simulink model "ADRC_IM"  (R2023b)
settings: Solver=FixedStepAuto  StartTime=0  StopTime=5  FixedStep=Ts  RelTol=1e-3
InitFcn:
  | Parameters_v7_1;
  | Parameters;
  | Sim;
StartFcn:
  | Parameters_v7_1;
  | Parameters;
  | Sim;
values from neighbouring files (symbols this model uses):
  F = 0.01    [Parameters_v7_2.m]
  J = 1.662    [Parameters_v7_2.m]
  ki_m = ((wc_m^2)*J)/(Kt)    [Parameters.m]
  kp_m = (2*damp*wc_m*J-F)/Kt    [Parameters.m]
  kr = Lm/Lr    (= 0.977464788732)    [Parameters_v7_2.m]
  Lm = 34.7e-3    (= 0.0347)    [Parameters_v7_2.m]
  p = 2    [Parameters_v7_2.m]
  r_sigma = Rs+kr^2*Rr    (= 0.304839730212)    [Parameters_v7_2.m]
  Rs = 0.087    [Parameters_v7_2.m]
  sf_nom = 0.973    [Parameters.m]    (also in Parameters_v7_2.m = 0.9)
  T_nom = 229    [Parameters_v7_2.m]
  t_sigma = sigma*Ls/r_sigma    (= 0.00518951984994)    [Parameters_v7_2.m]
  tr = Lr/Rr    (= 0.155701754386)    [Parameters_v7_2.m]
  Ts = 1e-6    (= 1e-06)    [Parameters.m]    (also in Parameters_v7_2.m = 5e-05)
  Tss = 1/fr    (= 2.5e-05)    [Parameters.m]
  Vdc = 780    [Parameters_v7_2.m]
undefined symbols (not defined in the file or in its folder): DiscIntNeverNeededParam, sigbuilder_block
libraries: spsAlphaBetaZerotoabcLib x2, slctrl_adaptive x1, slpidlib x1, spspowerguiLib x1
settings Model: Creator=Alvaro  LastModifiedBy=Selim
settings DebuggingCC: UnconnectedInputMsg=warning  UnconnectedOutputMsg=warning  UnconnectedLineMsg=warning
settings ModelReferenceCC: EnableRefExpFcnMdlSchedulingChecks=on
settings RTWCC: DLArmComputeVersion=19.05

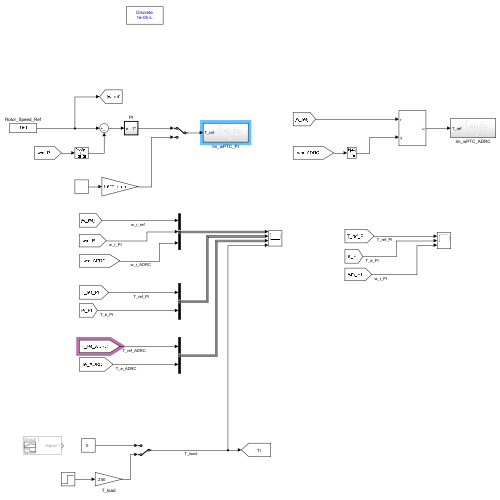
[thumbnail: Simulink's stored preview of the top-level diagram]
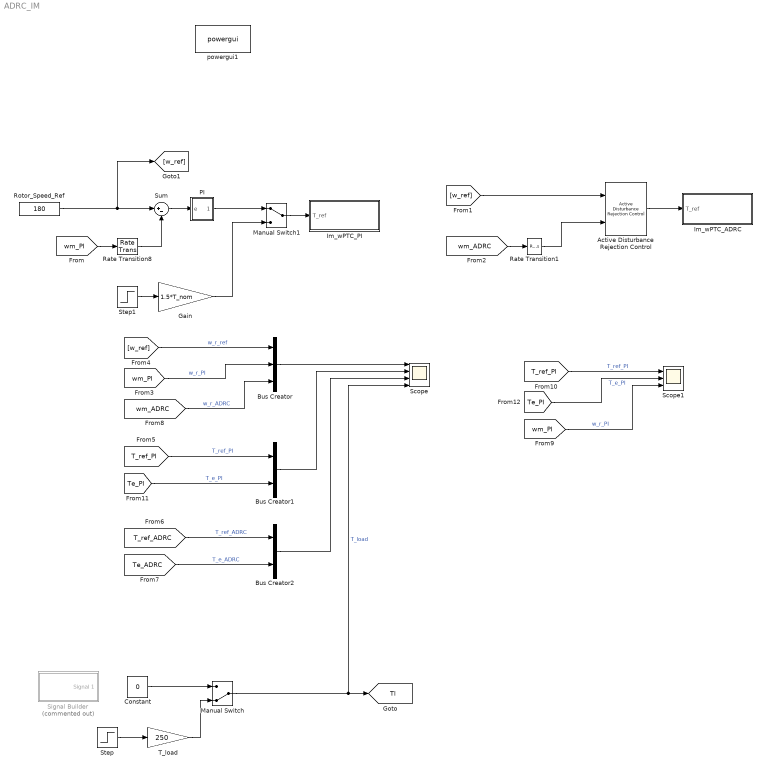
== system ADRC_IM ==
  Active Disturbance Rejection Control : slctrl_adaptive/Active Disturbance Rejection Control  time_domain=discrete-time  Ts=Ts  model_type=second-order  b0=b  wc=omega_C  wo=omega_O  x0=0  ulim_checkbox=on  umax=T_nom*1.5  umin=-T_nom*1.5  xhat_checkbox=off
      settings: LibrarySourceBlock=slctrlblks/Adaptive Control/Active Disturbance Rejection Control
  Bus Creator : BusCreator  Inputs=3
  Bus Creator1 : BusCreator  Inputs=2
  Bus Creator2 : BusCreator  Inputs=2
  Constant : Constant  Value=0
  Gain : Gain  Gain=1.5*T_nom
  Im_wPTC_ADRC : Subsystem
  Im_wPTC_PI : Subsystem
  Manual Switch : ManualSwitch  CurrentSetting=0
  Manual Switch1 : ManualSwitch
  PI : Subsystem  TreatAsAtomicUnit=on  SystemSampleTime=Tss
  Rate Transition1 : RateTransition  Integrity=off  Deterministic=off  InitialCondition=120  OutPortSampleTime=Ts
  Rate Transition8 : RateTransition  Integrity=off  Deterministic=off  InitialCondition=120  OutPortSampleTime=Ts
  Rotor_Speed_Ref : Constant  Value=180
  Scope : Scope  NumInputPorts=4
  Scope1 : Scope  NumInputPorts=3
  Signal Builder : Subsystem  Tag=STV Subsys  Commented=on  LoadFcn=sigbuilder_block('load');  StartFcn=sigbuilder_block('start');  StopFcn=sigbuilder_block('stop');  ClipboardFcn=sigbuilder_block('clipboard');  mask(Sigbuilder block){tuvar=[0:10]}
      mask help: Simulink:masks:SigbuilderBlock_MD
      mask init:
      | if ~strcmp(get_param(bdroot(gcbh),'SimulationStatus'),'stopped') tuvar = sigbuilder_block('maskInit'); end
      settings: CopyFcn=sigbuilder_block('copy');  DeleteFcn=sigbuilder_block('delete');  ModelCloseFcn=sigbuilder_block('modelClose');  PreSaveFcn=sigbuilder_block('preSave');  PauseFcn=sigbuilder_block('pause');  ContinueFcn=sigbuilder_block('continue');  NameChangeFcn=sigbuilder_block('namechange');  OpenFcn=sigbuilder_block('open',[437.25 153 550.5 359.25 ]);  CloseFcn=sigbuilder_block('close');
      mask Display: plot(0, 0, 100, 100,[2, 2, 32, 32, 2], [68, 8, 8, 68, 68],[32, 2], [38, 38], [32, 19, 2],[53, 60, 44], [32, 17, 17, 2],[16, 16, 31, 31]);txt = getActiveGroup(gcbh);text(2, 100, txt,'verticalAlignment', 'top');
  Step : Step  Time=1.5  SampleTime=0
  Step1 : Step  Time=0.5  SampleTime=0
  Sum : Sum  Inputs=|+-
  T_load : Gain  Gain=250
  powergui1 : spspowerguiLib/powergui  Priority=1  SimulationMode=Discrete  SampleTime=Ts  frequency=60  Iterations=50  frequencyindice=60  Pbase=100e6  ErrMax=1e-4  UnitsV=kV  UnitsW=MW  buscounter=0  FunctionMessages=off  echomessages=off  EnableUseOfTLC=off  CurrentSourceSwitches=off  DisableSnubberDevices=off  DisableRonSwitches=off  DisableVfSwitches=off  DisplayEquations=off  AutomaticDiscreteSolvers=off  SolverType=Tustin/Backward Euler (TBE)  Interpol=off  ExternalGateDelay=off  methode=off  Ts=100  x0status=blocks  SPID=off  SwTol=0  HookPort=off  NonlinearTolerance=1e-4  nMaxIteration=100  ContinueOnMaxIteration=off  RestoreLinks=warning  ResistiveCurrentMeasurement=off  Frange=[0:2:500]  Ylog=off  Xlog=on  ShowGrid=off  save=off  variable=ZData  structure=0  ZoomFFT=off  StartTime=0.0  cycles=1  DisplayStyle=1  fundamental=60  FreqAxis=off  MaxFrequency=1000  frequencyindicesteady=1  RmsSteady=1  display=off
  tag scope: Tl=global
  wires:
  [wm_PI] -> Rate Transition8/1
  Rotor_Speed_Ref/1 -> [w_ref], Sum/1
  Sum/1 -> PI/1(e)
  Constant/1 -> Manual Switch/1
  Manual Switch/1 -> Scope/4, [Tl]  "T_load"
  Step/1 -> T_load/1
  T_load/1 -> Manual Switch/2
  [w_ref] -> Bus Creator/1  "w_r_ref"
  [wm_PI] -> Bus Creator/2  "w_r_PI"
  Bus Creator/1 -> Scope/1
  [T_ref_PI] -> Bus Creator1/1  "T_ref_PI"
  Bus Creator1/1 -> Scope/2
  Rate Transition8/1 -> Sum/2
  PI/1(T*) -> Manual Switch1/1
  Active Disturbance Rejection Control/1 -> Im_wPTC_ADRC/1(T_ref)
  [wm_ADRC] -> Rate Transition1/1
  Rate Transition1/1 -> Active Disturbance Rejection Control/2
  [Te_ADRC] -> Bus Creator2/2  "T_e_ADRC"
  Bus Creator2/1 -> Scope/3
  [Te_PI] -> Bus Creator1/2  "T_e_PI"
  [T_ref_ADRC] -> Bus Creator2/1  "T_ref_ADRC"
  Step1/1 -> Gain/1
  Gain/1 -> Manual Switch1/2
  Manual Switch1/1 -> Im_wPTC_PI/1(T_ref)
  [w_ref] -> Active Disturbance Rejection Control/1
  [wm_ADRC] -> Bus Creator/3  "w_r_ADRC"
  [wm_PI] -> Scope1/3  "w_r_PI"
  [T_ref_PI] -> Scope1/1  "T_ref_PI"
  [Te_PI] -> Scope1/2  "T_e_PI"

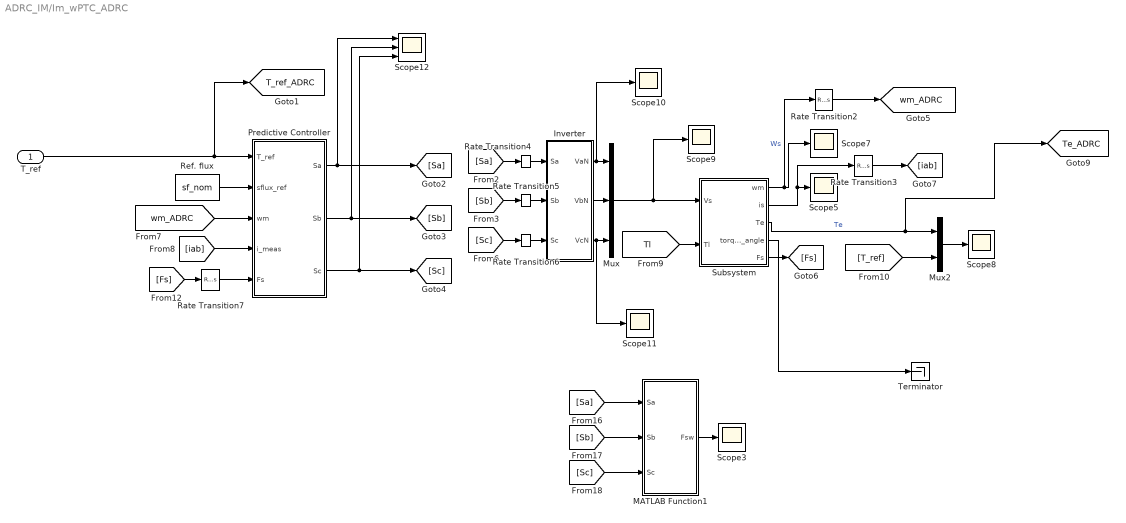
== system ADRC_IM/Im_wPTC_ADRC ==
  T_ref : Inport
  Inverter : Subsystem
  MATLAB Function1 : MATLAB Function  TreatAsAtomicUnit=on
  Mux : Mux  Inputs=3
  Mux2 : Mux  Inputs=2
  Predictive Controller : MATLAB Function  TreatAsAtomicUnit=on  SystemSampleTime=Tss
  Rate Transition2 : RateTransition  Integrity=off  Deterministic=off  InitialCondition=120  OutPortSampleTime=Tss
  Rate Transition3 : RateTransition  Integrity=off  Deterministic=off  InitialCondition=120  OutPortSampleTime=Tss
  Rate Transition4 : RateTransition  Integrity=off  Deterministic=off  InitialCondition=120  OutPortSampleTime=Ts
  Rate Transition5 : RateTransition  Integrity=off  Deterministic=off  InitialCondition=120  OutPortSampleTime=Ts
  Rate Transition6 : RateTransition  Integrity=off  Deterministic=off  InitialCondition=120  OutPortSampleTime=Ts
  Rate Transition7 : RateTransition  Integrity=off  Deterministic=off  InitialCondition=120  OutPortSampleTime=Tss
  Ref. flux : Constant  Value=sf_nom  SampleTime=Tss
  Scope{3,5,7..11} (7 alike) : Scope
  Scope12 : Scope  NumInputPorts=3
  Subsystem : Subsystem
  Terminator : Terminator
  tag scope: T_ref_ADRC=global, Te_ADRC=global, wm_ADRC=global
  wires:
  Subsystem/2(is) -> Rate Transition3/1, Scope5/1
  Rate Transition3/1 -> [iab]
  Rate Transition7/1 -> Predictive Controller/5(Fs)
  Inverter/3(VcN) -> Scope11/1, Mux/3
  Subsystem/4(torque_angle) -> Terminator/1
  Mux2/1 -> Scope8/1
  [Sb] -> Rate Transition5/1
  Predictive Controller/1(Sa) -> [Sa], Scope12/1
  Rate Transition6/1 -> Inverter/3(Sc)
  [Sa] -> MATLAB Function1/1(Sa)
  Subsystem/1(wm) -> Rate Transition2/1, Scope7/1  "Ws"
  [iab] -> Predictive Controller/4(i_meas)
  Ref. flux/1 -> Predictive Controller/2(sflux_ref)
  Mux/1 -> Scope9/1, Subsystem/1(Vs)
  Rate Transition4/1 -> Inverter/1(Sa)
  MATLAB Function1/1(Fsw) -> Scope3/1
  [Fs] -> Rate Transition7/1
  Subsystem/5(Fs) -> [Fs]
  Inverter/2(VbN) -> Mux/2
  Inverter/1(VaN) -> Scope10/1, Mux/1
  Rate Transition5/1 -> Inverter/2(Sb)
  [T_ref] -> Mux2/2
  Rate Transition2/1 -> [wm_ADRC]
  Predictive Controller/2(Sb) -> [Sb], Scope12/2
  [Sc] -> Rate Transition6/1
  Subsystem/3(Te) -> [Te_ADRC], Mux2/1  "Te"
  [Sc] -> MATLAB Function1/3(Sc)
  [wm_ADRC] -> Predictive Controller/3(wm)
  T_ref/1 -> [T_ref_ADRC], Predictive Controller/1(T_ref)
  Predictive Controller/3(Sc) -> [Sc], Scope12/3
  [Sb] -> MATLAB Function1/2(Sb)
  [Tl] -> Subsystem/2(Tl)
  [Sa] -> Rate Transition4/1

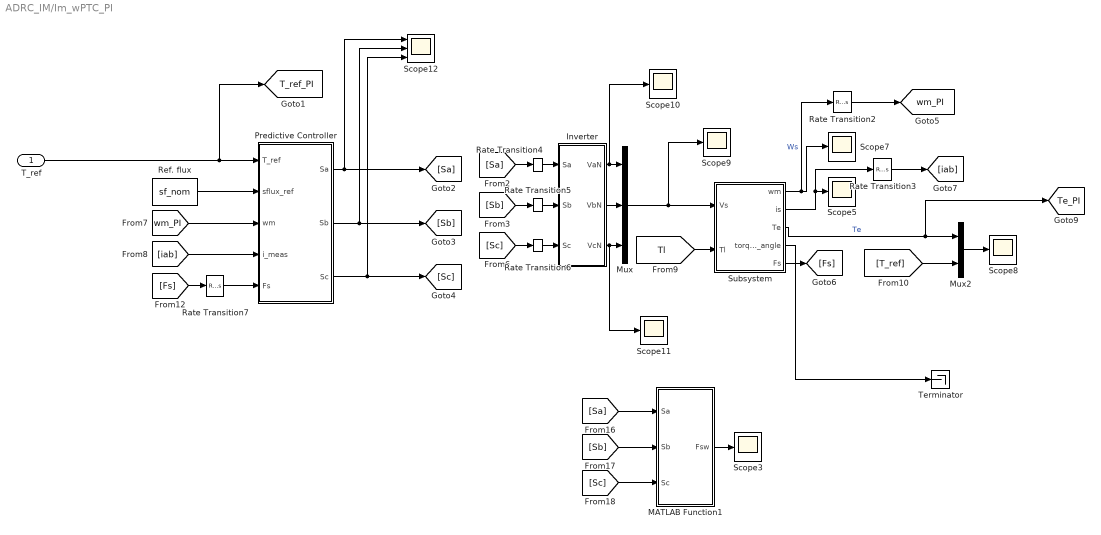
== system ADRC_IM/Im_wPTC_PI ==
  T_ref : Inport
  Inverter : Subsystem
  MATLAB Function1 : MATLAB Function  TreatAsAtomicUnit=on
  Mux : Mux  Inputs=3
  Mux2 : Mux  Inputs=2
  Predictive Controller : MATLAB Function  TreatAsAtomicUnit=on  SystemSampleTime=Tss
  Rate Transition2 : RateTransition  Integrity=off  Deterministic=off  InitialCondition=120  OutPortSampleTime=Tss
  Rate Transition3 : RateTransition  Integrity=off  Deterministic=off  InitialCondition=120  OutPortSampleTime=Tss
  Rate Transition4 : RateTransition  Integrity=off  Deterministic=off  InitialCondition=120  OutPortSampleTime=Ts
  Rate Transition5 : RateTransition  Integrity=off  Deterministic=off  InitialCondition=120  OutPortSampleTime=Ts
  Rate Transition6 : RateTransition  Integrity=off  Deterministic=off  InitialCondition=120  OutPortSampleTime=Ts
  Rate Transition7 : RateTransition  Integrity=off  Deterministic=off  InitialCondition=120  OutPortSampleTime=Tss
  Ref. flux : Constant  Value=sf_nom  SampleTime=Tss
  Scope{3,5,7..11} (7 alike) : Scope
  Scope12 : Scope  NumInputPorts=3
  Subsystem : Subsystem
  Terminator : Terminator
  tag scope: T_ref_PI=global, Te_PI=global, wm_PI=global
  wires:
  Subsystem/2(is) -> Rate Transition3/1, Scope5/1
  Rate Transition3/1 -> [iab]
  Rate Transition7/1 -> Predictive Controller/5(Fs)
  Inverter/3(VcN) -> Scope11/1, Mux/3
  Subsystem/4(torque_angle) -> Terminator/1
  Mux2/1 -> Scope8/1
  [Sb] -> Rate Transition5/1
  Predictive Controller/1(Sa) -> [Sa], Scope12/1
  Rate Transition6/1 -> Inverter/3(Sc)
  [Sa] -> MATLAB Function1/1(Sa)
  Subsystem/1(wm) -> Rate Transition2/1, Scope7/1  "Ws"
  [iab] -> Predictive Controller/4(i_meas)
  Ref. flux/1 -> Predictive Controller/2(sflux_ref)
  Mux/1 -> Scope9/1, Subsystem/1(Vs)
  Rate Transition4/1 -> Inverter/1(Sa)
  MATLAB Function1/1(Fsw) -> Scope3/1
  [Fs] -> Rate Transition7/1
  Subsystem/5(Fs) -> [Fs]
  Inverter/2(VbN) -> Mux/2
  Inverter/1(VaN) -> Scope10/1, Mux/1
  Rate Transition5/1 -> Inverter/2(Sb)
  [T_ref] -> Mux2/2
  Rate Transition2/1 -> [wm_PI]
  Predictive Controller/2(Sb) -> [Sb], Scope12/2
  [Sc] -> Rate Transition6/1
  Subsystem/3(Te) -> [Te_PI], Mux2/1  "Te"
  [Sc] -> MATLAB Function1/3(Sc)
  [wm_PI] -> Predictive Controller/3(wm)
  T_ref/1 -> [T_ref_PI], Predictive Controller/1(T_ref)
  Predictive Controller/3(Sc) -> [Sc], Scope12/3
  [Sb] -> MATLAB Function1/2(Sb)
  [Tl] -> Subsystem/2(Tl)
  [Sa] -> Rate Transition4/1

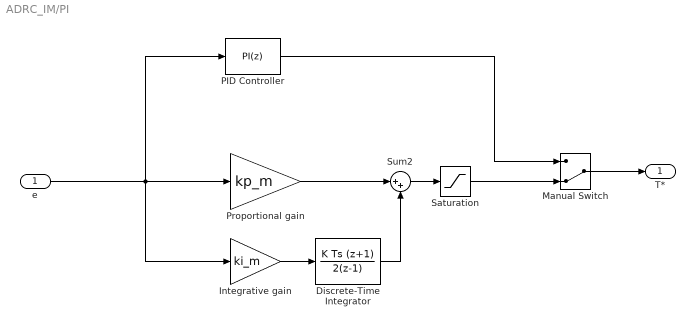
== system ADRC_IM/PI ==
  e : Inport
  Discrete-Time Integrator : DiscreteIntegrator  IntegratorMethod=Integration: Trapezoidal  SampleTime=-1  LimitOutput=on  UpperSaturationLimit=T_nom*1.5  LowerSaturationLimit=-T_nom*1.5  ICPrevOutput=DiscIntNeverNeededParam  ICPrevScaledInput=DiscIntNeverNeededParam
  Integrative gain : Gain  Gain=ki_m
  Manual Switch : ManualSwitch  CurrentSetting=0
  PID Controller : slpidlib/PID Controller  Controller=PI  Form=Parallel  TimeDomain=Discrete-time  UseExternalTs=off  SampleTime=-1  IntegratorMethod=Forward Euler  FilterMethod=Forward Euler  ControllerParametersSource=internal  P=kp_m  I=ki_m  UseKiTs=off  D=0  N=100  UseFilter=on  TunerSelectOption=Transfer Function Based (PID Tuner App)  InitialConditionSource=internal  InitialConditionForIntegrator=0  InitialConditionForFilter=0  DifferentiatorICPrevScaledInput=0  ExternalReset=none  TrackingMode=off  Kt=1  LimitOutput=on  SatLimitsSource=internal  UpperSaturationLimit=T_nom*1.5  LowerSaturationLimit=-T_nom*1.5  LinearizeAsGain=on  AntiWindupMode=clamping  Kb=1  LimitIntegrator=off  UpperIntegratorSaturationLimit=inf  LowerIntegratorSaturationLimit=-inf  POutMin=[]  POutMax=[]  IOutMin=[]  IOutMax=[]  DOutMin=[]  DOutMax=[]  NOutMin=[]  NOutMax=[]  SumOutMin=[]  SumOutMax=[]  SaturationOutMin=[]  SaturationOutMax=[]  PParamMin=[]  PParamMax=[]  IParamMin=[]  IParamMax=[]  DParamMin=[]  DParamMax=[]  NParamMin=[]  NParamMax=[]  KbParamMin=[]  KbParamMax=[]  KtParamMin=[]  KtParamMax=[]  KbOutMin=[]  KbOutMax=[]  KtOutMin=[]  KtOutMax=[]  IntegratorOutMin=[]  IntegratorOutMax=[]  FilterOutMin=[]  FilterOutMax=[]  SumI1OutMin=[]  SumI1OutMax=[]  SumI2OutMin=[]  SumI2OutMax=[]  SumI3OutMin=[]  SumI3OutMax=[]  SumI4OutMin=[]  SumI4OutMax=[]  SumDOutMin=[]  SumDOutMax=[]  DifferentiatorOutMin=[]  DifferentiatorOutMax=[]  FilterDiffOutCoefMin=[]  FilterDiffOutCoefMax=[]  ReciprocalOutMin=[]  ReciprocalOutMax=[]  SumDenOutMin=[]  SumDenOutMax=[]  SumNumOutMin=[]  SumNumOutMax=[]  DivideOutMin=[]  DivideOutMax=[]  UdiffTsProdOutMin=[]  UdiffTsProdOutMax=[]  NTsProdOutMin=[]  NTsProdOutMax=[]  UintegralTsProdOutMin=[]  UintegralTsProdOutMax=[]  UngainTsProdOutMin=[]  UngainTsProdOutMax=[]  ClampingZeroOutDataTypeStr=Inherit: Inherit via back propagation  ClampingZeroOutMin=[]  ClampingZeroOutMax=[]  FilterDenConstantOutDataTypeStr=Inherit: Inherit via back propagation  FilterDenConstantOutMin=[]  FilterDenConstantOutMax=[]  PCopyOutDataTypeStr=Inherit: Inherit via back propagation  PCopyOutMin=[]  PCopyOutMax=[]  NCopyOutDataTypeStr=Inherit: Inherit via back propagation  NCopyOutMin=[]  NCopyOutMax=[]  IntegratorContinuousStateAttributes=''  IntegratorStateMustResolveToSignalObject=off  IntegratorRTWStateStorageClass=Auto  FilterContinuousStateAttributes=''  FilterStateMustResolveToSignalObject=off  FilterRTWStateStorageClass=Auto  ParallelPVariant=InternalParameters  IdealPVariant=Disabled  IVariant=InternalParameters  DVariant=Disabled  IntegratorVariant=Discrete  SatVariant=Enabled  AWVariant=DiscClampingParallel  PCopyVariant=Disabled  TRVariant=Disabled  FdbkBlocksVariant=Forward  IdealPFdbkVariant=Disabled  SatFdbkVariant=Disabled  DerivativeFilterVariant=Disabled  NVariant=Disabled  NCopyVariant=Disabled_SignalSpec  FilterICVariant=Disabled  IntegratorICVariant=InternalICs  ExternalResetVariant=Disabled  TRSumVariant=Passthrough  SumFdbkVariant=Disabled  SumVariant=Sum_PI  TsampFilterVariant=InternalTs  TsampNgainVariant=Passthrough  TsampIntegralVariant=Disabled_SignalSpec  ExternalSaturationOutDataTypeStr=Inherit: Same as second input
  Proportional gain : Gain  Gain=kp_m
  Saturation : Saturate  UpperLimit=T_nom*1.5  LowerLimit=-T_nom*1.5
  Sum2 : Sum  Inputs=|++
  T* : Outport  VectorParamsAs1DForOutWhenUnconnected=off
  wires:
  e/1 -> PID Controller/1, Integrative gain/1, Proportional gain/1
  Sum2/1 -> Saturation/1
  Proportional gain/1 -> Sum2/1
  Saturation/1 -> Manual Switch/2
  Integrative gain/1 -> Discrete-Time Integrator/1
  Discrete-Time Integrator/1 -> Sum2/2
  Manual Switch/1 -> T*/1
  PID Controller/1 -> Manual Switch/1

== system ADRC_IM/Signal Builder ==
  Demux : Demux  Tag=STV Demux  Outputs=1
      settings: DisplayOption=none
  FromWs : FromWorkspace  Tag=STV FromWs  VariableName=tuvar
      SigBuilderData=|
      | common.afterFinalStr = 'Extrapolate'
      | common.sampleTime = 0
      | dataSet.timeRange = [0 10]
      | dataSet.name = 'Group 1'
      | sbobj.Groups.Name = 'Group 1'
      | sbobj.Groups.Signals.Name = 'Signal 1'
      | sbobj.Groups.Signals.XData = [0 1.5 1.5 2.02 2.02 3 3 4 4 10]
      | sbobj.Groups.Signals.YData = [0 0 100 100 229 229 150 150 50 50]
  Signal 1 : Outport  Tag=STV Outport  VectorParamsAs1DForOutWhenUnconnected=off
  wires:
  Demux/1 -> Signal 1/1
  FromWs/1 -> Demux/1

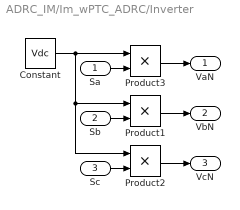
== system ADRC_IM/Im_wPTC_ADRC/Inverter ==
  Sa : Inport
  Sb : Inport  Port=2
  Sc : Inport  Port=3
  Constant : Constant  Value=Vdc
  Product1 : Product  RndMeth=Zero
  Product2 : Product  RndMeth=Zero
  Product3 : Product  RndMeth=Zero
  VaN : Outport  VectorParamsAs1DForOutWhenUnconnected=off
  VbN : Outport  Port=2  VectorParamsAs1DForOutWhenUnconnected=off
  VcN : Outport  Port=3  VectorParamsAs1DForOutWhenUnconnected=off
  wires:
  Product3/1 -> VaN/1
  Product1/1 -> VbN/1
  Sa/1 -> Product3/2
  Constant/1 -> Product3/1, Product1/1, Product2/1
  Sb/1 -> Product1/2
  Product2/1 -> VcN/1
  Sc/1 -> Product2/2

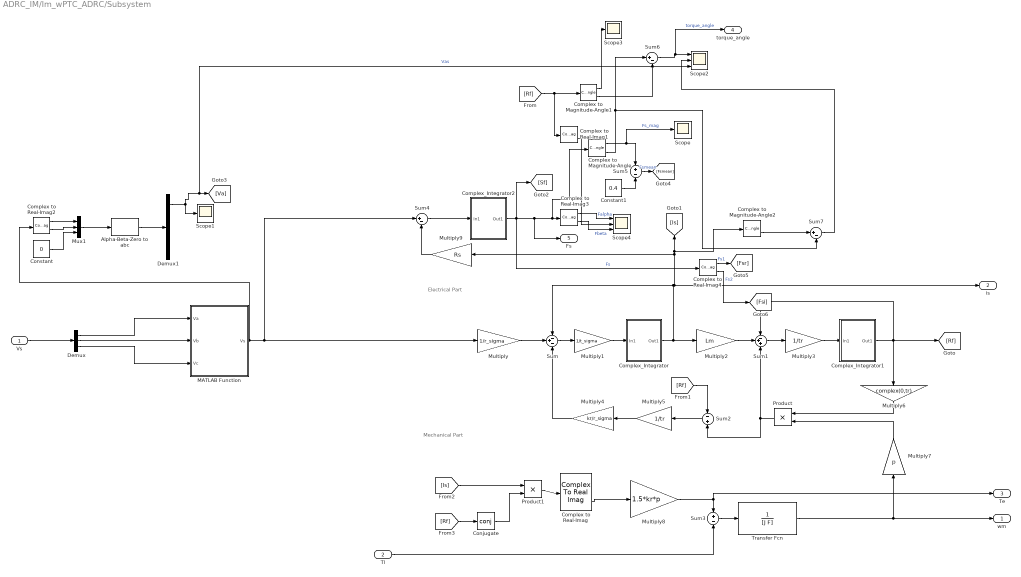
== system ADRC_IM/Im_wPTC_ADRC/Subsystem ==
  note: Mechanical Part
  note: Electrical Part
  Vs : Inport
  Tl : Inport  Port=2
  Alpha-Beta-Zero to abc : spsAlphaBetaZerotoabcLib/Alpha-Beta-Zero to abc
  Complex to Magnitude-Angle : ComplexToMagnitudeAngle
  Complex to Magnitude-Angle1 : ComplexToMagnitudeAngle
  Complex to Magnitude-Angle2 : ComplexToMagnitudeAngle
  Complex to Real-Imag{,1..4} (5 alike) : ComplexToRealImag
  Complex_Integrator : Subsystem
  Complex_Integrator1 : Subsystem
  Complex_Integrator2 : Subsystem
  Conjugate : Math  Operator=conj  SignedPower=on  RndMeth=Zero
  Constant : Constant  Value=0
  Constant1 : Constant  Value=0.4
  Demux : Demux  Outputs=3
  Demux1 : Demux  Outputs=3
  MATLAB Function : MATLAB Function  TreatAsAtomicUnit=on
  Multiply : Gain  Gain=1/r_sigma
  Multiply1 : Gain  Gain=1/t_sigma
  Multiply2 : Gain  Gain=Lm
  Multiply3 : Gain  Gain=1/tr
  Multiply4 : Gain  Gain=kr/r_sigma
  Multiply5 : Gain  Gain=1/tr
  Multiply6 : Gain  Gain=complex(0,tr)
  Multiply7 : Gain  Gain=p
  Multiply8 : Gain  Gain=1.5*kr*p
  Multiply9 : Gain  Gain=Rs
  Mux1 : Mux  Inputs=3
  Product : Product
  Product1 : Product
  Scope : Scope
  Scope1 : Scope
  Scope2 : Scope  NumInputPorts=3
  Scope3 : Scope
  Scope4 : Scope  NumInputPorts=3
  Sum : Sum  Inputs=-+-
  Sum1 : Sum  Inputs=-++
  Sum2 : Sum  Inputs=-+
  Sum3 : Sum  Inputs=+-
  Sum4 : Sum  Inputs=|+-
  Sum5 : Sum  Inputs=+-
  Sum6 : Sum  Inputs=|+-
  Sum7 : Sum  Inputs=|+-
  Transfer Fcn : TransferFcn  Denominator=[J F]
  wm : Outport
  is : Outport  Port=2
  Te : Outport  Port=3
  torque_angle : Outport  Port=4
  Fs : Outport  Port=5
  wires:
  [Is] -> Product1/1
  Multiply1/1 -> Complex_Integrator/1(In1)
  Multiply4/1 -> Sum/3
  Multiply3/1 -> Complex_Integrator1/1(In1)
  Sum1/1 -> Multiply3/1
  Complex to Real-Imag/2 -> Multiply8/1
  Complex_Integrator1/1(Out1) -> Sum1/1, [Rf], Multiply6/1
  Tl/1 -> Sum3/2
  Conjugate/1 -> Product1/2
  Multiply7/1 -> Product/2
  Multiply8/1 -> Sum3/1, Te/1
  Multiply2/1 -> Sum1/2
  Multiply/1 -> Sum/2
  Multiply6/1 -> Product/1
  Product/1 -> Sum2/2, Sum1/3
  Multiply5/1 -> Multiply4/1
  Sum2/1 -> Multiply5/1
  Transfer Fcn/1 -> wm/1, Multiply7/1
  Sum/1 -> Multiply1/1
  [Rf] -> Conjugate/1
  Product1/1 -> Complex to Real-Imag/1
  Sum3/1 -> Transfer Fcn/1
  [Rf] -> Sum2/1
  Sum4/1 -> Complex_Integrator2/1(In1)
  Complex_Integrator2/1(Out1) -> Complex to Real-Imag4/1, Fs/1, Complex to Magnitude-Angle/1, Complex to Real-Imag3/1, [Sf]  "Fs"
  Multiply9/1 -> Sum4/2
  Complex_Integrator/1(Out1) -> Multiply2/1, is/1, [Is], Complex to Magnitude-Angle2/1, Multiply9/1, Sum/1
  MATLAB Function/1(Vs) -> Complex to Real-Imag2/1, Sum4/1, Multiply/1
  Vs/1 -> Demux/1
  Demux/1 -> MATLAB Function/1(Va)
  Demux/2 -> MATLAB Function/2(Vb)
  Demux/3 -> MATLAB Function/3(Vc)
  Constant/1 -> Mux1/3
  Alpha-Beta-Zero to abc/1 -> Demux1/1
  Mux1/1 -> Alpha-Beta-Zero to abc/1
  Complex to Real-Imag2/2 -> Mux1/2
  Complex to Real-Imag2/1 -> Mux1/1
  Demux1/1 -> Scope2/3, [Va], Scope1/1  "Vas"
  Complex to Magnitude-Angle/1 -> Scope/1, Sum5/1  "Fs_mag"
  Constant1/1 -> Sum5/2
  Sum5/1 -> [Fsmean]  "Fsmean"
  [Rf] -> Complex to Real-Imag1/1, Complex to Magnitude-Angle1/1
  Complex to Magnitude-Angle1/2 -> Sum6/2
  Complex to Magnitude-Angle/2 -> Sum7/2, Sum6/1
  Sum6/1 -> torque_angle/1, Scope2/1  "torque_angle"
  Complex to Magnitude-Angle1/1 -> Scope3/1
  Complex to Magnitude-Angle2/2 -> Sum7/1
  Sum7/1 -> Scope2/2
  Complex to Real-Imag3/2 -> Scope4/3  "Fbeta"
  Complex to Real-Imag1/2 -> Scope4/2
  Complex to Real-Imag3/1 -> Scope4/1  "Falpha"
  Complex to Real-Imag4/2 -> [Fsi]  "Fs2"
  Complex to Real-Imag4/1 -> [Fsr]  "Fs1"

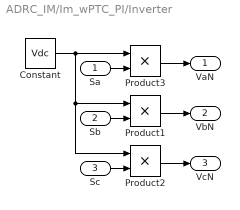
== system ADRC_IM/Im_wPTC_PI/Inverter ==
  Sa : Inport
  Sb : Inport  Port=2
  Sc : Inport  Port=3
  Constant : Constant  Value=Vdc
  Product1 : Product  RndMeth=Zero
  Product2 : Product  RndMeth=Zero
  Product3 : Product  RndMeth=Zero
  VaN : Outport  VectorParamsAs1DForOutWhenUnconnected=off
  VbN : Outport  Port=2  VectorParamsAs1DForOutWhenUnconnected=off
  VcN : Outport  Port=3  VectorParamsAs1DForOutWhenUnconnected=off
  wires:
  Product3/1 -> VaN/1
  Product1/1 -> VbN/1
  Sa/1 -> Product3/2
  Constant/1 -> Product3/1, Product1/1, Product2/1
  Sb/1 -> Product1/2
  Product2/1 -> VcN/1
  Sc/1 -> Product2/2

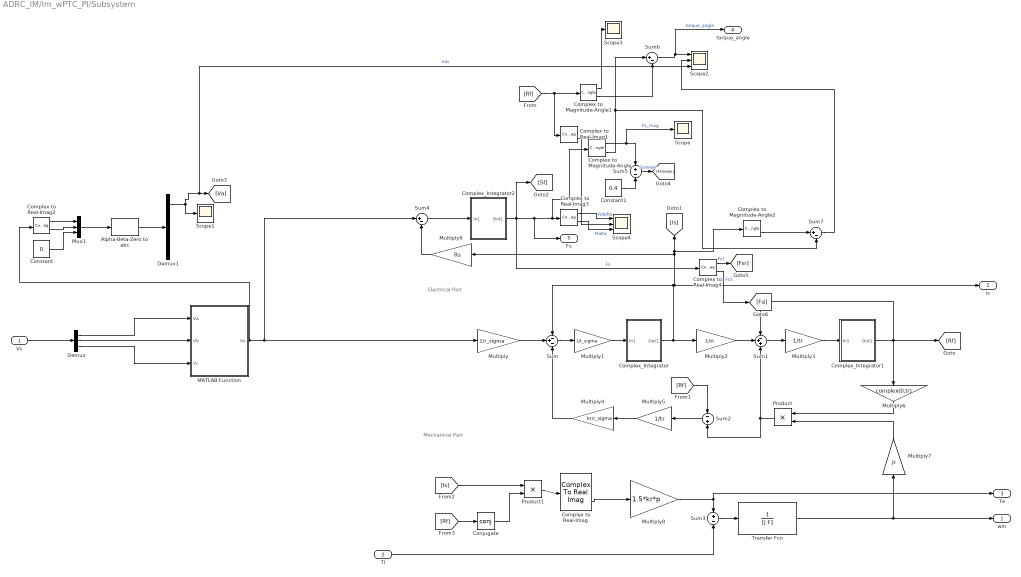
== system ADRC_IM/Im_wPTC_PI/Subsystem ==
  note: Mechanical Part
  note: Electrical Part
  Vs : Inport
  Tl : Inport  Port=2
  Alpha-Beta-Zero to abc : spsAlphaBetaZerotoabcLib/Alpha-Beta-Zero to abc
  Complex to Magnitude-Angle : ComplexToMagnitudeAngle
  Complex to Magnitude-Angle1 : ComplexToMagnitudeAngle
  Complex to Magnitude-Angle2 : ComplexToMagnitudeAngle
  Complex to Real-Imag{,1..4} (5 alike) : ComplexToRealImag
  Complex_Integrator : Subsystem
  Complex_Integrator1 : Subsystem
  Complex_Integrator2 : Subsystem
  Conjugate : Math  Operator=conj  SignedPower=on  RndMeth=Zero
  Constant : Constant  Value=0
  Constant1 : Constant  Value=0.4
  Demux : Demux  Outputs=3
  Demux1 : Demux  Outputs=3
  MATLAB Function : MATLAB Function  TreatAsAtomicUnit=on
  Multiply : Gain  Gain=1/r_sigma
  Multiply1 : Gain  Gain=1/t_sigma
  Multiply2 : Gain  Gain=Lm
  Multiply3 : Gain  Gain=1/tr
  Multiply4 : Gain  Gain=kr/r_sigma
  Multiply5 : Gain  Gain=1/tr
  Multiply6 : Gain  Gain=complex(0,tr)
  Multiply7 : Gain  Gain=p
  Multiply8 : Gain  Gain=1.5*kr*p
  Multiply9 : Gain  Gain=Rs
  Mux1 : Mux  Inputs=3
  Product : Product
  Product1 : Product
  Scope : Scope
  Scope1 : Scope
  Scope2 : Scope  NumInputPorts=3
  Scope3 : Scope
  Scope4 : Scope  NumInputPorts=3
  Sum : Sum  Inputs=-+-
  Sum1 : Sum  Inputs=-++
  Sum2 : Sum  Inputs=-+
  Sum3 : Sum  Inputs=+-
  Sum4 : Sum  Inputs=|+-
  Sum5 : Sum  Inputs=+-
  Sum6 : Sum  Inputs=|+-
  Sum7 : Sum  Inputs=|+-
  Transfer Fcn : TransferFcn  Denominator=[J F]
  wm : Outport
  is : Outport  Port=2
  Te : Outport  Port=3
  torque_angle : Outport  Port=4
  Fs : Outport  Port=5
  wires:
  [Is] -> Product1/1
  Multiply1/1 -> Complex_Integrator/1(In1)
  Multiply4/1 -> Sum/3
  Multiply3/1 -> Complex_Integrator1/1(In1)
  Sum1/1 -> Multiply3/1
  Complex to Real-Imag/2 -> Multiply8/1
  Complex_Integrator1/1(Out1) -> Sum1/1, [Rf], Multiply6/1
  Tl/1 -> Sum3/2
  Conjugate/1 -> Product1/2
  Multiply7/1 -> Product/2
  Multiply8/1 -> Sum3/1, Te/1
  Multiply2/1 -> Sum1/2
  Multiply/1 -> Sum/2
  Multiply6/1 -> Product/1
  Product/1 -> Sum2/2, Sum1/3
  Multiply5/1 -> Multiply4/1
  Sum2/1 -> Multiply5/1
  Transfer Fcn/1 -> wm/1, Multiply7/1
  Sum/1 -> Multiply1/1
  [Rf] -> Conjugate/1
  Product1/1 -> Complex to Real-Imag/1
  Sum3/1 -> Transfer Fcn/1
  [Rf] -> Sum2/1
  Sum4/1 -> Complex_Integrator2/1(In1)
  Complex_Integrator2/1(Out1) -> Complex to Real-Imag4/1, Fs/1, Complex to Magnitude-Angle/1, Complex to Real-Imag3/1, [Sf]  "Fs"
  Multiply9/1 -> Sum4/2
  Complex_Integrator/1(Out1) -> Multiply2/1, is/1, [Is], Complex to Magnitude-Angle2/1, Multiply9/1, Sum/1
  MATLAB Function/1(Vs) -> Complex to Real-Imag2/1, Sum4/1, Multiply/1
  Vs/1 -> Demux/1
  Demux/1 -> MATLAB Function/1(Va)
  Demux/2 -> MATLAB Function/2(Vb)
  Demux/3 -> MATLAB Function/3(Vc)
  Constant/1 -> Mux1/3
  Alpha-Beta-Zero to abc/1 -> Demux1/1
  Mux1/1 -> Alpha-Beta-Zero to abc/1
  Complex to Real-Imag2/2 -> Mux1/2
  Complex to Real-Imag2/1 -> Mux1/1
  Demux1/1 -> Scope2/3, [Va], Scope1/1  "Vas"
  Complex to Magnitude-Angle/1 -> Scope/1, Sum5/1  "Fs_mag"
  Constant1/1 -> Sum5/2
  Sum5/1 -> [Fsmean]  "Fsmean"
  [Rf] -> Complex to Real-Imag1/1, Complex to Magnitude-Angle1/1
  Complex to Magnitude-Angle1/2 -> Sum6/2
  Complex to Magnitude-Angle/2 -> Sum7/2, Sum6/1
  Sum6/1 -> torque_angle/1, Scope2/1  "torque_angle"
  Complex to Magnitude-Angle1/1 -> Scope3/1
  Complex to Magnitude-Angle2/2 -> Sum7/1
  Sum7/1 -> Scope2/2
  Complex to Real-Imag3/2 -> Scope4/3  "Fbeta"
  Complex to Real-Imag1/2 -> Scope4/2
  Complex to Real-Imag3/1 -> Scope4/1  "Falpha"
  Complex to Real-Imag4/2 -> [Fsi]  "Fs2"
  Complex to Real-Imag4/1 -> [Fsr]  "Fs1"

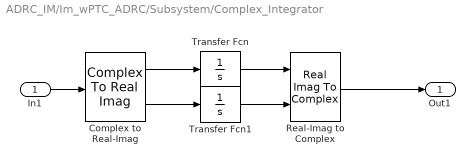
== system ADRC_IM/Im_wPTC_ADRC/Subsystem/Complex_Integrator ==
  In1 : Inport
  Complex to Real-Imag : ComplexToRealImag
  Real-Imag to Complex : RealImagToComplex
  Transfer Fcn : TransferFcn  Denominator=[1 0]
  Transfer Fcn1 : TransferFcn  Denominator=[1 0]
  Out1 : Outport
  wires:
  In1/1 -> Complex to Real-Imag/1
  Complex to Real-Imag/1 -> Transfer Fcn/1
  Complex to Real-Imag/2 -> Transfer Fcn1/1
  Transfer Fcn/1 -> Real-Imag to Complex/1
  Transfer Fcn1/1 -> Real-Imag to Complex/2
  Real-Imag to Complex/1 -> Out1/1

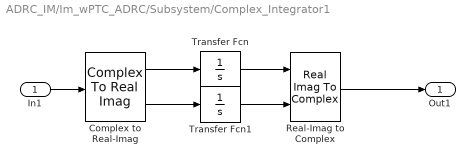
== system ADRC_IM/Im_wPTC_ADRC/Subsystem/Complex_Integrator1 ==
  In1 : Inport
  Complex to Real-Imag : ComplexToRealImag
  Real-Imag to Complex : RealImagToComplex
  Transfer Fcn : TransferFcn  Denominator=[1 0]
  Transfer Fcn1 : TransferFcn  Denominator=[1 0]
  Out1 : Outport
  wires:
  In1/1 -> Complex to Real-Imag/1
  Complex to Real-Imag/1 -> Transfer Fcn/1
  Complex to Real-Imag/2 -> Transfer Fcn1/1
  Transfer Fcn/1 -> Real-Imag to Complex/1
  Transfer Fcn1/1 -> Real-Imag to Complex/2
  Real-Imag to Complex/1 -> Out1/1

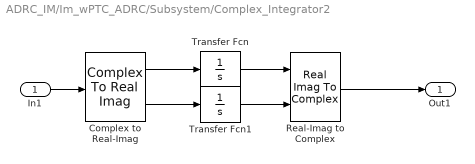
== system ADRC_IM/Im_wPTC_ADRC/Subsystem/Complex_Integrator2 ==
  In1 : Inport
  Complex to Real-Imag : ComplexToRealImag
  Real-Imag to Complex : RealImagToComplex
  Transfer Fcn : TransferFcn  Denominator=[1 0]
  Transfer Fcn1 : TransferFcn  Denominator=[1 0]
  Out1 : Outport
  wires:
  In1/1 -> Complex to Real-Imag/1
  Complex to Real-Imag/1 -> Transfer Fcn/1
  Complex to Real-Imag/2 -> Transfer Fcn1/1
  Transfer Fcn/1 -> Real-Imag to Complex/1
  Transfer Fcn1/1 -> Real-Imag to Complex/2
  Real-Imag to Complex/1 -> Out1/1

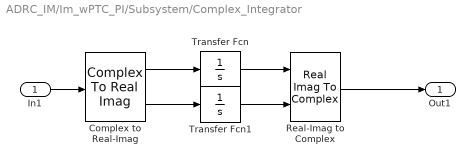
== system ADRC_IM/Im_wPTC_PI/Subsystem/Complex_Integrator ==
  In1 : Inport
  Complex to Real-Imag : ComplexToRealImag
  Real-Imag to Complex : RealImagToComplex
  Transfer Fcn : TransferFcn  Denominator=[1 0]
  Transfer Fcn1 : TransferFcn  Denominator=[1 0]
  Out1 : Outport
  wires:
  In1/1 -> Complex to Real-Imag/1
  Complex to Real-Imag/1 -> Transfer Fcn/1
  Complex to Real-Imag/2 -> Transfer Fcn1/1
  Transfer Fcn/1 -> Real-Imag to Complex/1
  Transfer Fcn1/1 -> Real-Imag to Complex/2
  Real-Imag to Complex/1 -> Out1/1

== system ADRC_IM/Im_wPTC_PI/Subsystem/Complex_Integrator1 ==
  In1 : Inport
  Complex to Real-Imag : ComplexToRealImag
  Real-Imag to Complex : RealImagToComplex
  Transfer Fcn : TransferFcn  Denominator=[1 0]
  Transfer Fcn1 : TransferFcn  Denominator=[1 0]
  Out1 : Outport
  wires:
  In1/1 -> Complex to Real-Imag/1
  Complex to Real-Imag/1 -> Transfer Fcn/1
  Complex to Real-Imag/2 -> Transfer Fcn1/1
  Transfer Fcn/1 -> Real-Imag to Complex/1
  Transfer Fcn1/1 -> Real-Imag to Complex/2
  Real-Imag to Complex/1 -> Out1/1

== system ADRC_IM/Im_wPTC_PI/Subsystem/Complex_Integrator2 ==
  In1 : Inport
  Complex to Real-Imag : ComplexToRealImag
  Real-Imag to Complex : RealImagToComplex
  Transfer Fcn : TransferFcn  Denominator=[1 0]
  Transfer Fcn1 : TransferFcn  Denominator=[1 0]
  Out1 : Outport
  wires:
  In1/1 -> Complex to Real-Imag/1
  Complex to Real-Imag/1 -> Transfer Fcn/1
  Complex to Real-Imag/2 -> Transfer Fcn1/1
  Transfer Fcn/1 -> Real-Imag to Complex/1
  Transfer Fcn1/1 -> Real-Imag to Complex/2
  Real-Imag to Complex/1 -> Out1/1

== matlab function ADRC_IM/Im_wPTC_ADRC/Subsystem/MATLAB Function ==
  data: Va input; Vs output; Vb input; Vc input
function Vs = fcn(Va,Vb,Vc)

a=complex(cos(2*pi/3),sin(2*pi/3)); 
Vs =(2/3)*(Va+(a*Vb)+((a^2)*Vc)) ;

== matlab function ADRC_IM/Im_wPTC_PI/Subsystem/MATLAB Function ==
  data: Va input; Vs output; Vb input; Vc input
function Vs = fcn(Va,Vb,Vc)

a=complex(cos(2*pi/3),sin(2*pi/3)); 
Vs =(2/3)*(Va+(a*Vb)+((a^2)*Vc)) ;

== matlab function ADRC_IM/Im_wPTC_PI/Predictive Controller ==
  settings: updateMethod=DISCRETE  sampleTime=Tss
  data: T_ref input; sflux_ref input; wm input; i_meas input; Sa output size=1; Sb output size=1; Sc output size=1; Fs input
function [Sa,Sb,Sc] = control(T_ref,sflux_ref,wm,i_meas,Fs)
 %global Ts Rs Lr Lm Ls p tr kr r_sigma t_sigma lambda v states
% Variables defined in the parameters file
 % global Ts Rs Lr Lm Ls p tr kr r_sigma t_sigma lambda v states
 % Sampling time of the predictive algorithm [s]% PI speed controller parameters
 % Sampling time of the predictive algorithm [s]
 Ts = 2.5e-5;
 % PI speed controller parameters
 %Kp = ; % Proportional gain
 %Ki = ; % Integrative gain
 % Machine parameters
 p = 2; % Pole pairs
 Lls =8e-4;
 Llr = 8e-4; 
  b=-2000*12.5;
  % b = -20;
 Lm=34.7e-3; % Magnetizing inductance [H]
 Ls = Lm+Lls; % Stator inductance [H]
 Lr = Lm+Llr; % Rotor inductance [H]
 Rs = 0.087; % Stator resistance [Ohm]
 Rr = 0.228; % Rotor resistance [Ohm]
 % Lm = 0.2687; % Magnetizing inductance [H]
 % Ls = 0.2815; % Stator inductance [H]
 % Lr = 0.2815; % Rotor inductance [H]
 % Rs = 2.845; % Stator resistance [Ohm]
 % Rr = 2.413; % Rotor resistance [Ohm]
 % DC-link voltage [V]
 %V=460 
 % Vdc = 780; %if is necessary change Vdc
 Vdc = 540;
 % Auxiliary constants
 ts = Ls/Rs;
 tr = Lr/Rr;
 sigma = 1-(((Lm)^2)/(Lr*Ls));
 kr = Lm/Lr;
 r_sigma = Rs+kr^2*Rr;
 t_sigma = sigma*Ls/r_sigma;
  sigma_s=1/(Ls*Lr-(Lm)^2);
 % Weighting factor for the cost function of PTC
 lambda = 600;
 % Voltage vectors
 v0 = 0;
 v1 = 2/3*Vdc;
 v2 = 1/3*Vdc + 1j*sqrt(3)/3*Vdc;
 v3 = -1/3*Vdc + 1j*sqrt(3)/3*Vdc;
 v4 = -2/3*Vdc;
 v5 = -1/3*Vdc - 1j*sqrt(3)/3*Vdc;
 v6 = 1/3*Vdc - 1j*sqrt(3)/3*Vdc;
 v7 = 0;
 v = [v0 v1 v2 v3 v4 v5 v6 v7];
% Switching states
 states = [0 0 0;1 0 0;1 1 0;0 1 0;0 1 1;0 0 1;1 0 1;1 1 1];
 persistent x_opt Fs1 i_estk F_estk
 if isempty(x_opt), x_opt = 1; end
 %if isempty(Fs), Fs = 10 + 10i*1; end
 if isempty(Fs1), Fs1 = 0 + 0i*1; end
 if isempty(i_estk), i_estk = 0 + 0i*1; end
 if isempty(F_estk), F_estk = 0 + 0i*1; end
 
 g=ones(1,8);
%% Full state observer for stator flux prediction
 i_est = (1-Ts*(sigma_s*(Rs*Lr+Rr*Ls)+1i*wm*p))*i_estk+Ts*sigma_s*(Rr-1i*Lr*p*wm)*...
 F_estk+Ts*v(x_opt)*sigma_s*Lr-2*b*Ts*(i_meas-i_estk);
 F_est = F_estk + Ts*v(x_opt) - Rs*Ts*i_estk-b/(sigma_s*Lr)*Ts*(i_meas-i_estk); 
 
%  % Stator flux estimate
 Fs1 = Fs1 + Ts*(v(x_opt) - Rs*i_meas);
 % Rotor flux estimate
 Fr = Lr/Lm*F_est+i_meas*(Lm-Lr*Ls/Lm);
 g_opt = 1e10;
 %g=zeros(1,8);
 for i = 1:8
 % i-th voltage vector for current prediction
 v_o1 = v(i);
 % Stator flux prediction at instant k+1
 Fsp1 = F_est + Ts*v_o1 - Rs*Ts*i_meas;
 % Stator current prediction at instant k+1
 Isp1 = (1+Ts/t_sigma)*i_meas+Ts/(t_sigma+Ts)*...
 (1/r_sigma*((kr/tr-kr*1i*wm*p)*Fr+v_o1));
 % Torque prediction at instant k+1
 Tp1 = 3/2*p*imag(conj(Fsp1)*Isp1);
 % Cost function
 Fsw=abs(states(i,1)-states(x_opt,1))+abs(states(i,2)-states(x_opt,2))+abs(states(i,3)-states(x_opt,3));
 g(i) = abs(T_ref - Tp1)+ lambda*abs(sflux_ref-abs(Fsp1))+0.5*Fsw;
 end
 
 for i = 1:8
 if (g(i)<g_opt)
 g_opt = g(i);
 x_opt = i;
 end
 end
 
 F_estk=F_est;
i_estk=i_est;
 %**************************************
 % Optimization
 %[~, x_opt] = min(g);
 % Output switching states
 Sa = states(x_opt,1);
 Sb = states(x_opt,2);
 Sc = states(x_opt,3);

== matlab function ADRC_IM/Im_wPTC_ADRC/MATLAB Function1 ==
  data: Sa input; Fsw output; Sb input; Sc input
function Fsw  = Fswitching(Sa,Sb,Sc)
 Ts=25e-6;
 persistent Nswa Nswb Nswc timer Sa_old Sb_old Sc_old Fsw_old
 if isempty(Nswa), Nswa = 0; end
 if isempty(Nswb), Nswb = 0; end
 if isempty(Nswc), Nswc = 0; end
 if isempty(timer), timer = 0; end
 if isempty(Sa_old), Sa_old = 0; end
 if isempty(Sb_old), Sb_old = 0; end
 if isempty(Sc_old), Sc_old = 0; end
 if isempty(Fsw_old), Fsw_old = 0; end
 
 
 if(timer<0.5)
     timer=timer+Ts;
     Nswa = Nswa+abs(Sa-Sa_old);
     Nswb = Nswb+abs(Sb-Sb_old);
     Nswc = Nswc+abs(Sc-Sc_old);
     Fsw=Fsw_old;
 else
     Fsw=(Nswa+Nswb+Nswc)/(2*3*0.5);
     timer=Ts;
     Nswa=0;
     Nswb=0;
     Nswc=0;
 end
  

 
Sa_old = Sa;
Sb_old = Sb;
Sc_old = Sc;
Fsw_old=Fsw;

== matlab function ADRC_IM/Im_wPTC_PI/MATLAB Function1 ==
  data: Sa input; Fsw output; Sb input; Sc input
function Fsw  = Fswitching(Sa,Sb,Sc)
 Ts=25e-6;
 persistent Nswa Nswb Nswc timer Sa_old Sb_old Sc_old Fsw_old
 if isempty(Nswa), Nswa = 0; end
 if isempty(Nswb), Nswb = 0; end
 if isempty(Nswc), Nswc = 0; end
 if isempty(timer), timer = 0; end
 if isempty(Sa_old), Sa_old = 0; end
 if isempty(Sb_old), Sb_old = 0; end
 if isempty(Sc_old), Sc_old = 0; end
 if isempty(Fsw_old), Fsw_old = 0; end
 
 
 if(timer<0.5)
     timer=timer+Ts;
     Nswa = Nswa+abs(Sa-Sa_old);
     Nswb = Nswb+abs(Sb-Sb_old);
     Nswc = Nswc+abs(Sc-Sc_old);
     Fsw=Fsw_old;
 else
     Fsw=(Nswa+Nswb+Nswc)/(2*3*0.5);
     timer=Ts;
     Nswa=0;
     Nswb=0;
     Nswc=0;
 end
  

 
Sa_old = Sa;
Sb_old = Sb;
Sc_old = Sc;
Fsw_old=Fsw;

== matlab function ADRC_IM/Im_wPTC_ADRC/Predictive Controller ==
  settings: updateMethod=DISCRETE  sampleTime=Tss
  data: T_ref input; sflux_ref input; wm input; i_meas input; Sa output size=1; Sb output size=1; Sc output size=1; Fs input
function [Sa,Sb,Sc] = control(T_ref,sflux_ref,wm,i_meas,Fs)
 %global Ts Rs Lr Lm Ls p tr kr r_sigma t_sigma lambda v states
% Variables defined in the parameters file
 % global Ts Rs Lr Lm Ls p tr kr r_sigma t_sigma lambda v states
 % Sampling time of the predictive algorithm [s]% PI speed controller parameters
 % Sampling time of the predictive algorithm [s]
 Ts = 2.5e-5;
 % PI speed controller parameters
 %Kp = ; % Proportional gain
 %Ki = ; % Integrative gain
 % Machine parameters
 p = 2; % Pole pairs
 Lls =8e-4;
 Llr = 8e-4; 
  b=-2000*12.5;
  % b = -20;
 Lm=34.7e-3; % Magnetizing inductance [H]
 Ls = Lm+Lls; % Stator inductance [H]
 Lr = Lm+Llr; % Rotor inductance [H]
 Rs = 0.087; % Stator resistance [Ohm]
 Rr = 0.228; % Rotor resistance [Ohm]
 % Lm = 0.2687; % Magnetizing inductance [H]
 % Ls = 0.2815; % Stator inductance [H]
 % Lr = 0.2815; % Rotor inductance [H]
 % Rs = 2.845; % Stator resistance [Ohm]
 % Rr = 2.413; % Rotor resistance [Ohm]
 % DC-link voltage [V]
 %V=460 
 % Vdc = 780; %if is necessary change Vdc
 Vdc = 540;
 % Auxiliary constants
 ts = Ls/Rs;
 tr = Lr/Rr;
 sigma = 1-(((Lm)^2)/(Lr*Ls));
 kr = Lm/Lr;
 r_sigma = Rs+kr^2*Rr;
 t_sigma = sigma*Ls/r_sigma;
  sigma_s=1/(Ls*Lr-(Lm)^2);
 % Weighting factor for the cost function of PTC
 lambda = 600;
 % Voltage vectors
 v0 = 0;
 v1 = 2/3*Vdc;
 v2 = 1/3*Vdc + 1j*sqrt(3)/3*Vdc;
 v3 = -1/3*Vdc + 1j*sqrt(3)/3*Vdc;
 v4 = -2/3*Vdc;
 v5 = -1/3*Vdc - 1j*sqrt(3)/3*Vdc;
 v6 = 1/3*Vdc - 1j*sqrt(3)/3*Vdc;
 v7 = 0;
 v = [v0 v1 v2 v3 v4 v5 v6 v7];
% Switching states
 states = [0 0 0;1 0 0;1 1 0;0 1 0;0 1 1;0 0 1;1 0 1;1 1 1];
 persistent x_opt Fs1 i_estk F_estk
 if isempty(x_opt), x_opt = 1; end
 %if isempty(Fs), Fs = 10 + 10i*1; end
 if isempty(Fs1), Fs1 = 0 + 0i*1; end
 if isempty(i_estk), i_estk = 0 + 0i*1; end
 if isempty(F_estk), F_estk = 0 + 0i*1; end
 
 g=ones(1,8);
%% Full state observer for stator flux prediction
 i_est = (1-Ts*(sigma_s*(Rs*Lr+Rr*Ls)+1i*wm*p))*i_estk+Ts*sigma_s*(Rr-1i*Lr*p*wm)*...
 F_estk+Ts*v(x_opt)*sigma_s*Lr-2*b*Ts*(i_meas-i_estk);
 F_est = F_estk + Ts*v(x_opt) - Rs*Ts*i_estk-b/(sigma_s*Lr)*Ts*(i_meas-i_estk); 
 
%  % Stator flux estimate
 Fs1 = Fs1 + Ts*(v(x_opt) - Rs*i_meas);
 % Rotor flux estimate
 Fr = Lr/Lm*F_est+i_meas*(Lm-Lr*Ls/Lm);
 g_opt = 1e10;
 %g=zeros(1,8);
 for i = 1:8
 % i-th voltage vector for current prediction
 v_o1 = v(i);
 % Stator flux prediction at instant k+1
 Fsp1 = F_est + Ts*v_o1 - Rs*Ts*i_meas;
 % Stator current prediction at instant k+1
 Isp1 = (1+Ts/t_sigma)*i_meas+Ts/(t_sigma+Ts)*...
 (1/r_sigma*((kr/tr-kr*1i*wm*p)*Fr+v_o1));
 % Torque prediction at instant k+1
 Tp1 = 3/2*p*imag(conj(Fsp1)*Isp1);
 % Cost function
 Fsw=abs(states(i,1)-states(x_opt,1))+abs(states(i,2)-states(x_opt,2))+abs(states(i,3)-states(x_opt,3));
 g(i) = abs(T_ref - Tp1)+ lambda*abs(sflux_ref-abs(Fsp1))+0.5*Fsw;
 end
 
 for i = 1:8
 if (g(i)<g_opt)
 g_opt = g(i);
 x_opt = i;
 end
 end
 
 F_estk=F_est;
i_estk=i_est;
 %**************************************
 % Optimization
 %[~, x_opt] = min(g);
 % Output switching states
 Sa = states(x_opt,1);
 Sb = states(x_opt,2);
 Sc = states(x_opt,3);
